simulink model "VTOL_quadplane"  (R2026a)
settings: Solver=ode1  StopTime=120  FixedStep=1/60  MaxStep=0.01
undefined symbols (not defined in the file or in its folder): op_trim, params, Receive, Send
libraries: slpidlib x32, simulink_extras x11, simulink x2, aerolibfltsims x2, aerolibobsolete x1, sim3dlib x1, uavsim3dlib x1
(part 4 of 4)

== system VTOL_quadplane/Autopilot/Height Controller/Subsystem ==
  Constant : Constant  Commented=on  Value=params.trim_Inputs.delta_ele
  Constant1 : Constant  Commented=on  Value=params.trim_Inputs.delta_ail
  From : From  Commented=on  GotoTag=theta_rad  TagVisibility=global
  From1 : From  Commented=on  GotoTag=q_rads  TagVisibility=global
  From2 : From  Commented=on  GotoTag=phi_rad  TagVisibility=global
  From3 : From  Commented=on  GotoTag=p_rads  TagVisibility=global
  PID Controller : slpidlib/PID Controller  Commented=on  Controller=P  Form=Parallel  TimeDomain=Continuous-time  UseExternalTs=off  SampleTime=-1  IntegratorMethod=Forward Euler  FilterMethod=Forward Euler  ControllerParametersSource=internal  P=5.02  I=1  UseKiTs=off  D=0  UseExternalDerivativeSource=off  N=100  UseFilter=on  TunerSelectOption=Transfer Function Based (PID Tuner App)  InitialConditionSource=internal  InitialConditionForIntegrator=0  InitialConditionForFilter=0  DifferentiatorICPrevScaledInput=0  ExternalReset=none  TrackingMode=off  Kt=1  LimitOutput=off  SatLimitsSource=internal  UpperSaturationLimit=inf  LowerSaturationLimit=-inf  LinearizeAsGain=on  AntiWindupMode=none  Kb=1  LimitIntegrator=off  UpperIntegratorSaturationLimit=inf  LowerIntegratorSaturationLimit=-inf  POutMin=[]  POutMax=[]  IOutMin=[]  IOutMax=[]  DOutMin=[]  DOutMax=[]  NOutMin=[]  NOutMax=[]  SumOutMin=[]  SumOutMax=[]  SaturationOutMin=[]  SaturationOutMax=[]  PParamMin=[]  PParamMax=[]  IParamMin=[]  IParamMax=[]  DParamMin=[]  DParamMax=[]  NParamMin=[]  NParamMax=[]  KbParamMin=[]  KbParamMax=[]  KtParamMin=[]  KtParamMax=[]  KbOutMin=[]  KbOutMax=[]  KtOutMin=[]  KtOutMax=[]  IntegratorOutMin=[]  IntegratorOutMax=[]  FilterOutMin=[]  FilterOutMax=[]  SumI1OutMin=[]  SumI1OutMax=[]  SumI2OutMin=[]  SumI2OutMax=[]  SumI3OutMin=[]  SumI3OutMax=[]  SumI4OutMin=[]  SumI4OutMax=[]  SumDOutMin=[]  SumDOutMax=[]  DifferentiatorOutMin=[]  DifferentiatorOutMax=[]  FilterDiffOutCoefMin=[]  FilterDiffOutCoefMax=[]  ReciprocalOutMin=[]  ReciprocalOutMax=[]  SumDenOutMin=[]  SumDenOutMax=[]  SumNumOutMin=[]  SumNumOutMax=[]  DivideOutMin=[]  DivideOutMax=[]  UdiffTsProdOutMin=[]  UdiffTsProdOutMax=[]  NTsProdOutMin=[]  NTsProdOutMax=[]  UintegralTsProdOutMin=[]  UintegralTsProdOutMax=[]  UngainTsProdOutMin=[]  UngainTsProdOutMax=[]  ClampingZeroOutDataTypeStr=Inherit: Inherit via back propagation  ClampingZeroOutMin=[]  ClampingZeroOutMax=[]  FilterDenConstantOutDataTypeStr=Inherit: Inherit via back propagation  FilterDenConstantOutMin=[]  FilterDenConstantOutMax=[]  PCopyOutDataTypeStr=Inherit: Inherit via back propagation  PCopyOutMin=[]  PCopyOutMax=[]  NCopyOutDataTypeStr=Inherit: Inherit via back propagation  NCopyOutMin=[]  NCopyOutMax=[]  IntegratorContinuousStateAttributes=''  IntegratorStateMustResolveToSignalObject=off  IntegratorRTWStateStorageClass=Auto  FilterContinuousStateAttributes=''  FilterStateMustResolveToSignalObject=off  FilterRTWStateStorageClass=Auto  ParallelPVariant=InternalParameters  IdealPVariant=Disabled  IVariant=Disabled  DVariant=Disabled  IntegratorVariant=Disabled  SatVariant=Disabled  AWVariant=Disabled  PCopyVariant=Disabled  TRVariant=Disabled  FdbkBlocksVariant=Forward  IdealPFdbkVariant=Disabled  SatFdbkVariant=Disabled  DerivativeFilterVariant=Disabled  NVariant=Disabled  NCopyVariant=Disabled_SignalSpec  FilterICVariant=Disabled  IntegratorICVariant=Disabled  ExternalResetVariant=Disabled  TRSumVariant=Passthrough  SumFdbkVariant=Disabled  SumVariant=Passthrough_P  TsampFilterVariant=InternalTs  TsampNgainVariant=Passthrough  TsampIntegralVariant=Disabled_SignalSpec  ExternalSaturationOutDataTypeStr=Inherit: Same as second input  DerivativeSourceVariant=Disabled  PreIntVariant=InternalPreInt
  PID Controller1 : slpidlib/PID Controller  Commented=on  Controller=PID  Form=Parallel  TimeDomain=Continuous-time  UseExternalTs=off  SampleTime=-1  IntegratorMethod=Forward Euler  FilterMethod=Forward Euler  ControllerParametersSource=internal  P=-0.189  I=-1.81  UseKiTs=off  D=-0.00495  UseExternalDerivativeSource=off  N=100  UseFilter=on  TunerSelectOption=Transfer Function Based (PID Tuner App)  InitialConditionSource=internal  InitialConditionForIntegrator=0  InitialConditionForFilter=0  DifferentiatorICPrevScaledInput=0  ExternalReset=none  TrackingMode=off  Kt=1  LimitOutput=off  SatLimitsSource=internal  UpperSaturationLimit=inf  LowerSaturationLimit=-inf  LinearizeAsGain=on  AntiWindupMode=none  Kb=1  LimitIntegrator=off  UpperIntegratorSaturationLimit=inf  LowerIntegratorSaturationLimit=-inf  POutMin=[]  POutMax=[]  IOutMin=[]  IOutMax=[]  DOutMin=[]  DOutMax=[]  NOutMin=[]  NOutMax=[]  SumOutMin=[]  SumOutMax=[]  SaturationOutMin=[]  SaturationOutMax=[]  PParamMin=[]  PParamMax=[]  IParamMin=[]  IParamMax=[]  DParamMin=[]  DParamMax=[]  NParamMin=[]  NParamMax=[]  KbParamMin=[]  KbParamMax=[]  KtParamMin=[]  KtParamMax=[]  KbOutMin=[]  KbOutMax=[]  KtOutMin=[]  KtOutMax=[]  IntegratorOutMin=[]  IntegratorOutMax=[]  FilterOutMin=[]  FilterOutMax=[]  SumI1OutMin=[]  SumI1OutMax=[]  SumI2OutMin=[]  SumI2OutMax=[]  SumI3OutMin=[]  SumI3OutMax=[]  SumI4OutMin=[]  SumI4OutMax=[]  SumDOutMin=[]  SumDOutMax=[]  DifferentiatorOutMin=[]  DifferentiatorOutMax=[]  FilterDiffOutCoefMin=[]  FilterDiffOutCoefMax=[]  ReciprocalOutMin=[]  ReciprocalOutMax=[]  SumDenOutMin=[]  SumDenOutMax=[]  SumNumOutMin=[]  SumNumOutMax=[]  DivideOutMin=[]  DivideOutMax=[]  UdiffTsProdOutMin=[]  UdiffTsProdOutMax=[]  NTsProdOutMin=[]  NTsProdOutMax=[]  UintegralTsProdOutMin=[]  UintegralTsProdOutMax=[]  UngainTsProdOutMin=[]  UngainTsProdOutMax=[]  ClampingZeroOutDataTypeStr=Inherit: Inherit via back propagation  ClampingZeroOutMin=[]  ClampingZeroOutMax=[]  FilterDenConstantOutDataTypeStr=Inherit: Inherit via back propagation  FilterDenConstantOutMin=[]  FilterDenConstantOutMax=[]  PCopyOutDataTypeStr=Inherit: Inherit via back propagation  PCopyOutMin=[]  PCopyOutMax=[]  NCopyOutDataTypeStr=Inherit: Inherit via back propagation  NCopyOutMin=[]  NCopyOutMax=[]  IntegratorContinuousStateAttributes=''  IntegratorStateMustResolveToSignalObject=off  IntegratorRTWStateStorageClass=Auto  FilterContinuousStateAttributes=''  FilterStateMustResolveToSignalObject=off  FilterRTWStateStorageClass=Auto  ParallelPVariant=InternalParameters  IdealPVariant=Disabled  IVariant=InternalParameters  DVariant=InternalParameters  IntegratorVariant=Continuous  SatVariant=Disabled  AWVariant=Passthrough  PCopyVariant=Disabled  TRVariant=Disabled  FdbkBlocksVariant=Forward  IdealPFdbkVariant=Disabled  SatFdbkVariant=Disabled  DerivativeFilterVariant=ContFilter  NVariant=InternalParameters  NCopyVariant=Disabled  FilterICVariant=InternalICsFilter  IntegratorICVariant=InternalICs  ExternalResetVariant=Disabled  TRSumVariant=Passthrough  SumFdbkVariant=Disabled  SumVariant=Sum_PID  TsampFilterVariant=InternalTs  TsampNgainVariant=Passthrough  TsampIntegralVariant=Disabled_SignalSpec  ExternalSaturationOutDataTypeStr=Inherit: Same as second input  DerivativeSourceVariant=ErrorSignal  PreIntVariant=InternalPreInt
  PID Controller2 : slpidlib/PID Controller  Commented=on  Controller=P  Form=Parallel  TimeDomain=Continuous-time  UseExternalTs=off  SampleTime=-1  IntegratorMethod=Forward Euler  FilterMethod=Forward Euler  ControllerParametersSource=internal  P=5.02  I=1  UseKiTs=off  D=0  UseExternalDerivativeSource=off  N=100  UseFilter=on  TunerSelectOption=Transfer Function Based (PID Tuner App)  InitialConditionSource=internal  InitialConditionForIntegrator=0  InitialConditionForFilter=0  DifferentiatorICPrevScaledInput=0  ExternalReset=none  TrackingMode=off  Kt=1  LimitOutput=off  SatLimitsSource=internal  UpperSaturationLimit=inf  LowerSaturationLimit=-inf  LinearizeAsGain=on  AntiWindupMode=none  Kb=1  LimitIntegrator=off  UpperIntegratorSaturationLimit=inf  LowerIntegratorSaturationLimit=-inf  POutMin=[]  POutMax=[]  IOutMin=[]  IOutMax=[]  DOutMin=[]  DOutMax=[]  NOutMin=[]  NOutMax=[]  SumOutMin=[]  SumOutMax=[]  SaturationOutMin=[]  SaturationOutMax=[]  PParamMin=[]  PParamMax=[]  IParamMin=[]  IParamMax=[]  DParamMin=[]  DParamMax=[]  NParamMin=[]  NParamMax=[]  KbParamMin=[]  KbParamMax=[]  KtParamMin=[]  KtParamMax=[]  KbOutMin=[]  KbOutMax=[]  KtOutMin=[]  KtOutMax=[]  IntegratorOutMin=[]  IntegratorOutMax=[]  FilterOutMin=[]  FilterOutMax=[]  SumI1OutMin=[]  SumI1OutMax=[]  SumI2OutMin=[]  SumI2OutMax=[]  SumI3OutMin=[]  SumI3OutMax=[]  SumI4OutMin=[]  SumI4OutMax=[]  SumDOutMin=[]  SumDOutMax=[]  DifferentiatorOutMin=[]  DifferentiatorOutMax=[]  FilterDiffOutCoefMin=[]  FilterDiffOutCoefMax=[]  ReciprocalOutMin=[]  ReciprocalOutMax=[]  SumDenOutMin=[]  SumDenOutMax=[]  SumNumOutMin=[]  SumNumOutMax=[]  DivideOutMin=[]  DivideOutMax=[]  UdiffTsProdOutMin=[]  UdiffTsProdOutMax=[]  NTsProdOutMin=[]  NTsProdOutMax=[]  UintegralTsProdOutMin=[]  UintegralTsProdOutMax=[]  UngainTsProdOutMin=[]  UngainTsProdOutMax=[]  ClampingZeroOutDataTypeStr=Inherit: Inherit via back propagation  ClampingZeroOutMin=[]  ClampingZeroOutMax=[]  FilterDenConstantOutDataTypeStr=Inherit: Inherit via back propagation  FilterDenConstantOutMin=[]  FilterDenConstantOutMax=[]  PCopyOutDataTypeStr=Inherit: Inherit via back propagation  PCopyOutMin=[]  PCopyOutMax=[]  NCopyOutDataTypeStr=Inherit: Inherit via back propagation  NCopyOutMin=[]  NCopyOutMax=[]  IntegratorContinuousStateAttributes=''  IntegratorStateMustResolveToSignalObject=off  IntegratorRTWStateStorageClass=Auto  FilterContinuousStateAttributes=''  FilterStateMustResolveToSignalObject=off  FilterRTWStateStorageClass=Auto  ParallelPVariant=InternalParameters  IdealPVariant=Disabled  IVariant=Disabled  DVariant=Disabled  IntegratorVariant=Disabled  SatVariant=Disabled  AWVariant=Disabled  PCopyVariant=Disabled  TRVariant=Disabled  FdbkBlocksVariant=Forward  IdealPFdbkVariant=Disabled  SatFdbkVariant=Disabled  DerivativeFilterVariant=Disabled  NVariant=Disabled  NCopyVariant=Disabled_SignalSpec  FilterICVariant=Disabled  IntegratorICVariant=Disabled  ExternalResetVariant=Disabled  TRSumVariant=Passthrough  SumFdbkVariant=Disabled  SumVariant=Passthrough_P  TsampFilterVariant=InternalTs  TsampNgainVariant=Passthrough  TsampIntegralVariant=Disabled_SignalSpec  ExternalSaturationOutDataTypeStr=Inherit: Same as second input  DerivativeSourceVariant=Disabled  PreIntVariant=InternalPreInt
  PID Controller3 : slpidlib/PID Controller  Commented=on  Controller=PID  Form=Parallel  TimeDomain=Continuous-time  UseExternalTs=off  SampleTime=-1  IntegratorMethod=Forward Euler  FilterMethod=Forward Euler  ControllerParametersSource=internal  P=-0.189  I=-1.81  UseKiTs=off  D=-0.00495  UseExternalDerivativeSource=off  N=100  UseFilter=on  TunerSelectOption=Transfer Function Based (PID Tuner App)  InitialConditionSource=internal  InitialConditionForIntegrator=0  InitialConditionForFilter=0  DifferentiatorICPrevScaledInput=0  ExternalReset=none  TrackingMode=off  Kt=1  LimitOutput=off  SatLimitsSource=internal  UpperSaturationLimit=inf  LowerSaturationLimit=-inf  LinearizeAsGain=on  AntiWindupMode=none  Kb=1  LimitIntegrator=off  UpperIntegratorSaturationLimit=inf  LowerIntegratorSaturationLimit=-inf  POutMin=[]  POutMax=[]  IOutMin=[]  IOutMax=[]  DOutMin=[]  DOutMax=[]  NOutMin=[]  NOutMax=[]  SumOutMin=[]  SumOutMax=[]  SaturationOutMin=[]  SaturationOutMax=[]  PParamMin=[]  PParamMax=[]  IParamMin=[]  IParamMax=[]  DParamMin=[]  DParamMax=[]  NParamMin=[]  NParamMax=[]  KbParamMin=[]  KbParamMax=[]  KtParamMin=[]  KtParamMax=[]  KbOutMin=[]  KbOutMax=[]  KtOutMin=[]  KtOutMax=[]  IntegratorOutMin=[]  IntegratorOutMax=[]  FilterOutMin=[]  FilterOutMax=[]  SumI1OutMin=[]  SumI1OutMax=[]  SumI2OutMin=[]  SumI2OutMax=[]  SumI3OutMin=[]  SumI3OutMax=[]  SumI4OutMin=[]  SumI4OutMax=[]  SumDOutMin=[]  SumDOutMax=[]  DifferentiatorOutMin=[]  DifferentiatorOutMax=[]  FilterDiffOutCoefMin=[]  FilterDiffOutCoefMax=[]  ReciprocalOutMin=[]  ReciprocalOutMax=[]  SumDenOutMin=[]  SumDenOutMax=[]  SumNumOutMin=[]  SumNumOutMax=[]  DivideOutMin=[]  DivideOutMax=[]  UdiffTsProdOutMin=[]  UdiffTsProdOutMax=[]  NTsProdOutMin=[]  NTsProdOutMax=[]  UintegralTsProdOutMin=[]  UintegralTsProdOutMax=[]  UngainTsProdOutMin=[]  UngainTsProdOutMax=[]  ClampingZeroOutDataTypeStr=Inherit: Inherit via back propagation  ClampingZeroOutMin=[]  ClampingZeroOutMax=[]  FilterDenConstantOutDataTypeStr=Inherit: Inherit via back propagation  FilterDenConstantOutMin=[]  FilterDenConstantOutMax=[]  PCopyOutDataTypeStr=Inherit: Inherit via back propagation  PCopyOutMin=[]  PCopyOutMax=[]  NCopyOutDataTypeStr=Inherit: Inherit via back propagation  NCopyOutMin=[]  NCopyOutMax=[]  IntegratorContinuousStateAttributes=''  IntegratorStateMustResolveToSignalObject=off  IntegratorRTWStateStorageClass=Auto  FilterContinuousStateAttributes=''  FilterStateMustResolveToSignalObject=off  FilterRTWStateStorageClass=Auto  ParallelPVariant=InternalParameters  IdealPVariant=Disabled  IVariant=InternalParameters  DVariant=InternalParameters  IntegratorVariant=Continuous  SatVariant=Disabled  AWVariant=Passthrough  PCopyVariant=Disabled  TRVariant=Disabled  FdbkBlocksVariant=Forward  IdealPFdbkVariant=Disabled  SatFdbkVariant=Disabled  DerivativeFilterVariant=ContFilter  NVariant=InternalParameters  NCopyVariant=Disabled  FilterICVariant=InternalICsFilter  IntegratorICVariant=InternalICs  ExternalResetVariant=Disabled  TRSumVariant=Passthrough  SumFdbkVariant=Disabled  SumVariant=Sum_PID  TsampFilterVariant=InternalTs  TsampNgainVariant=Passthrough  TsampIntegralVariant=Disabled_SignalSpec  ExternalSaturationOutDataTypeStr=Inherit: Same as second input  DerivativeSourceVariant=ErrorSignal  PreIntVariant=InternalPreInt
  Saturation1 : Saturate  Commented=on  UpperLimit=deg2rad(25)  LowerLimit=-deg2rad(25)
  Saturation3 : Saturate  Commented=on  UpperLimit=deg2rad(25)  LowerLimit=-deg2rad(25)
  Sum{,1,4..5} (4 alike) : Sum  Commented=on  Inputs=|+-
  Sum3 : Sum  Commented=on  Inputs=++|
  Sum6 : Sum  Commented=on  Inputs=++|
  Transfer Fcn : TransferFcn  Commented=on  Denominator=[0.02 1]
  Transfer Fcn1 : TransferFcn  Commented=on  Denominator=[0.02 1]
  wires:
  Sum/1 -> PID Controller/1
  Saturation3/1 -> Sum4/1
  Saturation1/1 -> Sum/1
  Sum6/1 -> Transfer Fcn1/1
  PID Controller1/1 -> Sum3/2
  PID Controller2/1 -> Sum5/1
  Transfer Fcn1/1 -> ?
  From/1 -> Sum/2
  Constant/1 -> Sum3/1
  Transfer Fcn/1 -> ?
  From2/1 -> Sum4/2
  From3/1 -> Sum5/2
  Sum4/1 -> PID Controller2/1
  From1/1 -> Sum1/2
  Sum3/1 -> Transfer Fcn/1
  PID Controller3/1 -> Sum6/2
  Sum5/1 -> PID Controller3/1
  ? -> Saturation1/1
  PID Controller/1 -> Sum1/1
  ? -> Saturation3/1
  Constant1/1 -> Sum6/1
  Sum1/1 -> PID Controller1/1

== matlab function VTOL_quadplane/MATLAB Function1 ==
  settings: updateMethod=DISCRETE
  data: cruise_speed input; lambda output; mc_forward_speed output; cruise_altitude input; mc_speed input; speed input; height input; transition_speed input; mc_height output; fw_speed output; fw_height output; mode output; transition_height input
function [lambda, mc_forward_speed, mc_height, fw_speed, fw_height, mode] = mode_manager( ...
    cruise_speed, cruise_altitude, mc_speed, speed, height, transition_speed, transition_height)
%MODE_MANAGER  VTOL quadplane mission state machine.
%
%   0 = climb straight to transition_height
%   1 = hover at transition_height for HOVER_TIME before transitioning
%   2 = TRANSITION: lambda ramps 0->1, forward-speed target ramps 0->
%       transition_speed, AND altitude ramps transition_height->
%       cruise_altitude - ALL CONTINUOUSLY, no step inputs to any
%       controller, so nothing gets a derivative kick.
%   3 = COMPLETE FW: only entered once lambda has reached 1, the aircraft
%       has reached cruise_altitude, AND transition_speed has been
%       reached. MC path is given no active target here.

    persistent state timer lambda_state climb_timer speed_timer
    if isempty(state)
        state       = 0;
        timer       = 0;
        lambda_state = 0;
        climb_timer  = 0;
        speed_timer  = 0;
    end

    DT              = 1/100;  % [s] model's fixed step = 1/simulation time
    HOVER_TIME      = 0.5;    % [s] wait at transition altitude before ramping
    T_LAMBDA_RAMP   = 20.0;   % [s] total time for lambda to go 0->1, smoothly
    ALT_CLIMB_TIME  = 10.0;   % [s] time to climb from transition_height to cruise_altitude
    SPEED_RAMP_TIME = 5.0;   % [s] time to ramp forward-speed target to transition_speed
                              % (feeds the pitch PID - must NOT be a step)

    alt_target   = transition_height;  % defaults so they're defined on every path
    speed_target = 0;

    % ---- state transitions ----
    if state == 0 && height <= transition_height + 0.5
        state = 1;
        timer = 0;
    end

    if state == 1
        timer = timer + DT;
        if timer >= HOVER_TIME
            state       = 2;
            timer       = 0;
            climb_timer = 0;   % start all ramps together
            speed_timer = 0;
        end
    end

    if state == 2
        % ---- lambda ramp: smooth, continuous, no steps ----
        lambda_state = min(lambda_state + DT / T_LAMBDA_RAMP, 1);

        % ---- altitude ramp (smoothstep - no rate discontinuity) ----
        climb_timer = climb_timer + DT;
        fa = min(climb_timer / ALT_CLIMB_TIME, 1);
        sa = 3*fa^2 - 2*fa^3;
        alt_target = transition_height + sa * (cruise_altitude - transition_height);

        % ---- forward-speed ramp (smoothstep - no step into the PID) ----
        speed_timer = speed_timer + DT;
        fs = min(speed_timer / SPEED_RAMP_TIME, 1);
        ss = 3*fs^2 - 2*fs^3;
        speed_target = ss * transition_speed;

        % only lock into complete FW once ALL three are true
        if lambda_state >= 1 && height <= cruise_altitude + 0.5 && speed >= transition_speed
            state = 3;
        end
    end

    % ---- outputs ----
    if state == 0 || state == 1
        mc_forward_speed = 0;
        fw_speed         = 0;
        mc_height        = transition_height;
        fw_height        = transition_height;

    elseif state == 2
        mc_forward_speed = speed_target;   % ramped, not stepped
        fw_speed         = speed_target;
        mc_height        = alt_target;
        fw_height        = alt_target;

    else % state == 3 - complete FW, MC path given nothing to chase
        mc_forward_speed = 0;
        mc_height        = height;        % freeze - zero error, no MC climb command
        fw_speed         = cruise_speed;
        fw_height        = cruise_altitude;
    end

    lambda = lambda_state;
    mode   = state;
end

== matlab function VTOL_quadplane/MATLAB Function3 ==
  settings: updateMethod=DISCRETE
  data: cruise_speed input; lambda output; mc_forward_speed output; cruise_altitude input; mc_speed input; speed input; height input; transition_speed input; mc_height output; fw_speed output; fw_height output; mode output; transition_height input
function [lambda, mc_forward_speed, mc_height, fw_speed, fw_height, mode] = mode_manager( ...
    cruise_speed, cruise_altitude, mc_speed, speed, height, transition_speed, transition_height)

    persistent state hover_timer
    if isempty(state)
        state       = 0;   % 0 = climb, 1 = hover, 2 = transition/cruise
        hover_timer = 0;
    end

    DT         = 1/60;  % [s] model's fixed step
    HOVER_TIME = 5.0;   % [s]

    if state == 0 && height <= transition_height + 2
        state       = 1;
        hover_timer = 0;
    end

    if state == 1
        hover_timer = hover_timer + DT;
        if hover_timer >= HOVER_TIME
            state = 2;
        end
    end

    if state == 0 || state == 1
        mc_forward_speed = 0;
        mc_height        = transition_height;
        fw_speed         = 0;
        fw_height        = transition_height;
        lambda           = 0;
    else
        mc_forward_speed = cruise_speed;
        mc_height        = transition_height;
        fw_speed         = cruise_speed;
        fw_height        = transition_height;
        lambda           = 1;
    end

    mode = state;
end

== matlab function VTOL_quadplane/MATLAB Function4 ==
  settings: updateMethod=DISCRETE
  data: cruise_speed input; lambda output; mc_forward_speed output; cruise_altitude input; mc_speed input; speed input; height input; transition_speed input; mc_height output; fw_speed output; fw_height output; mode output; transition_height input
function [lambda, mc_forward_speed, mc_height, fw_speed, fw_height, mode] = mode_manager( ...
    cruise_speed, cruise_altitude, mc_speed, speed, height, transition_speed, transition_height)

    persistent state hover_timer lambda_state
    if isempty(state)
        state        = 0;   % 0 = climb, 1 = hover, 2 = transition/cruise
        hover_timer  = 0;
        lambda_state = 0;
    end

    DT         = 1/60;  % [s] model's fixed step
    HOVER_TIME = 5.0;   % [s]
    T_BLEND    = 6.0;   % [s] time for lambda to ramp 0 -> 1 - raise this
                        % to make the transition even gentler

    if state == 0 && height <= transition_height + 2
        state       = 1;
        hover_timer = 0;
    end

    if state == 1
        hover_timer = hover_timer + DT;
        if hover_timer >= HOVER_TIME
            state = 2;
        end
    end

    if state == 0 || state == 1
        mc_forward_speed = 0;
        mc_height        = transition_height;
        fw_speed         = 0;
        fw_height        = transition_height;
        lambda_state     = 0;
    else
        mc_forward_speed = cruise_speed;
        mc_height        = transition_height;
        fw_speed         = cruise_speed;
        fw_height        = transition_height;
        lambda_state     = min(lambda_state + DT / T_BLEND, 1);
    end

    lambda = lambda_state;
    mode   = state;
end

== matlab function VTOL_quadplane/MATLAB Function5 ==
  settings: updateMethod=DISCRETE
  data: cruise_speed input; lambda output; mc_forward_speed output; cruise_altitude input; mc_speed input; speed input; height input; transition_speed input; mc_height output; fw_speed output; fw_height output; mode output; transition_height input
function [lambda, mc_forward_speed, mc_height, fw_speed, fw_height, mode] = mode_manager( ...
    cruise_speed, cruise_altitude, mc_speed, speed, height, transition_speed, transition_height)

    persistent state timer lambda_state
    if isempty(state)
        state        = 0;   % 0 = climb, 1 = hover, 2 = ramp, 3 = cruise
        timer        = 0;
        lambda_state = 0;
    end

    DT         = 1/60;  % [s] model's fixed step
    HOVER_TIME = 5.0;   % [s] wait at transition altitude before ramping
    STEP_TIME  = 2.0;   % [s] between each 0.1 increment (10 steps x 1s = 10s)

    % ---- state transitions ----
    if state == 0 && height <= transition_height + 0.5
        state = 1;
        timer = 0;
    end

    if state == 1
        timer = timer + DT;
        if timer >= HOVER_TIME
            state = 2;
            timer = 0;
        end
    end

    if state == 2
        timer = timer + DT;
        if timer >= STEP_TIME
            timer        = 0;
            lambda_state = lambda_state + 0.1;
        end
        if lambda_state >= 1
            lambda_state = 1;
            state        = 3;
        end
    end

    if speed >= transition_speed
        lambda_state = 1;
        state        = 3;
    end

    % ---- outputs ----
    if state == 0 || state == 1
        mc_forward_speed = 0;
        fw_speed         = 0;
    else
        mc_forward_speed = cruise_speed;
        fw_speed         = cruise_speed;
    end

    mc_height = transition_height;
    fw_height = transition_height;
    lambda    = lambda_state;
    mode      = state;
end

== matlab function VTOL_quadplane/MATLAB Function6 ==
  settings: updateMethod=DISCRETE
  data: cruise_speed input; lambda output; mc_forward_speed output; cruise_altitude input; mc_speed input; speed input; height input; transition_speed input; mc_height output; fw_speed output; fw_height output; mode output; transition_height input
function [lambda, mc_forward_speed, mc_height, fw_speed, fw_height, mode] = mode_manager( ...
    cruise_speed, cruise_altitude, mc_speed, speed, height, transition_speed, transition_height)

    persistent state timer lambda_state
    if isempty(state)
        state        = 0;   % 0 = climb, 1 = hover, 2 = ramp, 3 = cruise
        timer        = 0;
        lambda_state = 0;
    end

    DT         = 1/600;  % [s] model's fixed step
    HOVER_TIME = 2.0;   % [s] wait at transition altitude before ramping
    STEP_TIME  = 1.0;   % [s] between each 0.1 increment (10 steps x 1s = 10s)

    % ---- state transitions ----
    if state == 0 && height <= transition_height + 0.5
        state = 1;
        timer = 0;
    end

    if state == 1
        timer = timer + DT;
        if timer >= HOVER_TIME
            state = 2;
            timer = 0;
        end
    end

    if state == 2
        timer = timer + DT;
        if timer >= STEP_TIME
            timer        = 0;
            lambda_state = lambda_state + 0.1;
        end
        if lambda_state >= 1
            lambda_state = 1;
            state        = 3;
        end
    end

    if speed >= transition_speed
        lambda_state = 1;
        state        = 3;
    end

    % ---- outputs ----
    if state == 0 || state == 1
        mc_forward_speed = 0;
        fw_speed         = 0;
    else
        mc_forward_speed = cruise_speed;
        fw_speed         = cruise_speed;
    end

    mc_height = transition_height;
    fw_height = transition_height;
    lambda    = lambda_state;
    mode      = state;
end

== matlab function VTOL_quadplane/MATLAB Function7 ==
  settings: updateMethod=DISCRETE
  data: cruise_speed input; lambda output; mc_forward_speed output; cruise_altitude input; mc_speed input; speed input; height input; transition_speed input; mc_height output; fw_speed output; fw_height output; mode output; transition_height input
function [lambda, mc_forward_speed, mc_height, fw_speed, fw_height, mode] = mode_manager( ...
    cruise_speed, cruise_altitude, mc_speed, speed, height, transition_speed, transition_height)

    persistent state timer lambda_state
    if isempty(state)
        state        = 0;   % 0 = climb, 1 = hover, 2 = ramp, 3 = cruise
        timer        = 0;
        lambda_state = 0;
    end

    DT         = 1/600;  % [s] model's fixed step
    HOVER_TIME = 0.5;   % [s] wait at transition altitude before ramping
    STEP_TIME  = 3.0;   % [s] between each 0.1 increment (10 steps x 1s = 10s)

    % ---- state transitions ----
    if state == 0 && height <= transition_height + 0.5
        state = 1;
        timer = 0;
    end

    if state == 1
        timer = timer + DT;
        if timer >= HOVER_TIME
            state = 2;
            timer = 0;
        end
    end

    if state == 2
        timer = timer + DT;
        if timer >= STEP_TIME
            timer        = 0;
            lambda_state = lambda_state + 0;
        end
        if lambda_state >= 1
            lambda_state = 1;
            state        = 3;
        end
    end

    if speed >= transition_speed
        lambda_state = 1+0;
        state        = 3;
    end

    % ---- outputs ----
    if state == 0 || state == 1
        mc_forward_speed = 0;
        fw_speed         = 0;
    else
        mc_forward_speed = cruise_speed;
        fw_speed         = cruise_speed;
        fw_height        = cruise_altitude;
    end

    mc_height = transition_height;
    fw_height = cruise_altitude;
    lambda    = lambda_state;
    mode      = state;
end

== matlab function VTOL_quadplane/Pusher Forces and Moments ==
  data: u input; F_fw output; M_fw output; params input
function [F_fw, M_fw] = pusher_forces_and_moments(u, params)


% Function to commute forces and moments contributed by the pusher motor
% FW_propulsion_data;
% Extracting appriopriate input
delta_T = u(1); % Throttle Input

% Thrust generated by pusher motor
T_pusher = interp1(params.fw.Throttle, params.fw.Thrust, delta_T, 'linear', 'extrap');
Q_pusher = interp1(params.fw.Throttle, params.fw.Torque, delta_T, 'linear', 'extrap');

% Clamp to zero to avoid negative thrust
T_pusher = max(T_pusher, 0);
Q_pusher = max(Q_pusher, 0);

F_fw = [T_pusher; 0 ; 0];    
% F_fw = F_fw';

% Moments generated by pusher motor
r_pusher = [0;0;0]; % pusher position


% Moment computation
% M_fw = cross(F_fw, r_pusher);
M_fw = cross(r_pusher, F_fw) + [Q_pusher; 0; 0];

% % M_fw = M';% + [Q_pusher, 0, 0];

end

== matlab function VTOL_quadplane/Motor Mixing/MATLAB Function ==
  data: Throttle input; sigma_1 output; roll input; pitch input; yaw input; sigma_2 output; sigma_3 output; sigma_4 output
function [sigma_1, sigma_2, sigma_3, sigma_4] = Motor_mapping(Throttle, roll, pitch, yaw)

Mix_mat = [1 , -1,  1,  1;
           1,   1, -1,  1;
           1,   1,  1, -1;
           1,  -1, -1, -1]; 

Inputs = [Throttle; roll; pitch; yaw]; %User inputs

sigma = Mix_mat*Inputs;

sigma_1 = sigma(1,:);
sigma_2 = sigma(2,:);
sigma_3 = sigma(3,:);
sigma_4 = sigma(4,:);

end

== matlab function VTOL_quadplane/Autopilot/MATLAB Function ==
  data: theta_c input; del_e output; theta input; q input; Va input; params input; zeta_theta input; theta_e_max input; delta_e_max input; kp_theta output; kd_theta output; omega_n_theta output; K_theta_DC output
function [del_e, kp_theta, kd_theta, omega_n_theta, K_theta_DC] = ...
    pitch_attitude_controller(theta_c, theta, q, Va, params, zeta_theta, theta_e_max, delta_e_max)
%PITCH_ATTITUDE_CONTROLLER  Pitch-attitude-hold autopilot (elevator channel).
%
%   Implements the successive-loop-closure pitch attitude hold loop from
%   Beard & McLain, "Small Unmanned Aircraft," Ch. 6, Sec. 6.4.1
%   (Fig. 6.15, Eqs. 6.18-6.23), using the a_theta1..a_theta3 coefficients
%   from Ch. 5 (Sec. 5.5) and the airframe parameters produced by Params1.m.
%
%   [del_e, kp_theta, kd_theta, omega_n_theta, K_theta_DC] = ...
%       pitch_attitude_controller(theta_c, theta, q, Va, params, ...
%                                  zeta_theta, theta_e_max, delta_e_max)
%
% INPUTS
%   theta_c      - commanded pitch angle                        [rad]
%   theta        - current pitch angle                          [rad]
%   q            - body-axis pitch rate                         [rad/s]
%   Va           - airspeed at which a_theta1..3 are evaluated  [m/s]
%                  (use the trim/nominal airspeed for a fixed-gain
%                  design, per the book; pass the instantaneous
%                  airspeed instead if you want simple gain scheduling)
%   params       - aircraft parameter struct from Params1.m
%   zeta_theta   - desired pitch-loop damping ratio (design choice, e.g. 0.707)
%   theta_e_max  - maximum expected pitch error, used to size kp_theta [rad]
%   delta_e_max  - elevator actuator saturation limit                 [rad]
%
% OUTPUTS
%   del_e          - commanded elevator deflection [rad], saturated to
%                    +/- delta_e_max
%   kp_theta       - proportional gain                 (Eq. 6.?, ahead of 6.19)
%   kd_theta       - derivative (rate) gain             (Eq. 6.22)
%   omega_n_theta  - resulting pitch-loop natural frequency (Eq. 6.21)
%   K_theta_DC     - inner-loop DC gain, theta -> theta_c (Eq. 6.23),
%                    needed by the outer altitude/airspeed-from-pitch loops
%
%   Note: kp_theta, kd_theta, omega_n_theta and K_theta_DC only depend on
%   Va and params/tuning choices, not on theta_c/theta/q. If you are
%   calling this every simulation step with a fixed Va, you are free to
%   compute the gains once offline and hard-code them instead.

% ---- unpack the physical parameters needed for a_theta1..3 ----
rho = params.constants.rho;      % air density                [kg/m^3]
c   = params.geometric.c;        % mean aerodynamic chord     [m]
S   = params.geometric.S;        % wing area                  [m^2]
Jy  = params.geometric.I_y;      % pitch moment of inertia    [kg.m^2]

Cm_alpha = params.aero.Cm_alpha; % pitching-moment slope wrt alpha
Cm_q     = params.aero.Cm_q;     % pitching-moment slope wrt pitch rate
Cm_de    = params.aero.Cm_de;    % pitching-moment slope wrt elevator

% ---- longitudinal short-period coefficients (Ch.5, Sec 5.5) ----
a_theta1 = -(rho*Va^2*c*S)/(2*Jy) * Cm_q * (c/(2*Va));
a_theta2 = -(rho*Va^2*c*S)/(2*Jy) * Cm_alpha;
a_theta3 =  (rho*Va^2*c*S)/(2*Jy) * Cm_de;

% ---- pitch-loop gain design (Eqs. 6.19-6.23) ----
kp_theta      = (delta_e_max/theta_e_max) * sign(a_theta3);
omega_n_theta = sqrt(a_theta2 + (delta_e_max/theta_e_max)*abs(a_theta3));
kd_theta      = (2*zeta_theta*omega_n_theta - a_theta1) / a_theta3;
K_theta_DC    = (kp_theta*a_theta3) / (a_theta2 + kp_theta*a_theta3);

% ---- pitch attitude-hold control law (output of the pitch loop) ----
del_e_unsat = kp_theta*(theta_c - theta) - kd_theta*q;

% ---- elevator actuator saturation ----
del_e = max(min(del_e_unsat, delta_e_max), -delta_e_max);

end

== matlab function VTOL_quadplane/Motor Mixing/MATLAB Function1 ==
  data: u input; Omega_1 output; Throttle input; Omega_2 output; RPM input; Omega_3 output; Omega_4 output
function [Omega_1, Omega_2, Omega_3, Omega_4] = RPM_from_throttle_percentage(u,Throttle, RPM)


% NED frame
% Extracting control inputs
sigma1       = u(1); % Rotor 1 Throttle %
sigma2       = u(2); % Rotor 2 Throttle %
sigma3       = u(3); % Rotor 3 Throttle %
sigma4       = u(4); % Rotor 4 Throttle %

% % Motor Positioning
% % [M1:FR, M2:FL, M3:RL, M4:RR]
% % spin direction = [CW:+1, CCW:-1]
% % Extracting motor positions
% r1 = params.prop.r1(:); %FR-CCW
% r2 = params.prop.r2(:); %RL-CCW
% r3 = params.prop.r3(:); %FL-CW
% r4 = params.prop.r4(:); %RR-CW

% throttle to RPM mapping
W1       = interp1(Throttle, RPM, sigma1, 'linear','extrap');
Omega_1  = (W1*2*pi/60)^2;

W2       = interp1(Throttle, RPM, sigma2, 'linear','extrap');
Omega_2  = (W2*2*pi/60)^2;

W3       = interp1(Throttle, RPM, sigma3, 'linear','extrap');
Omega_3  = (W3*2*pi/60)^2;

W4       = interp1(Throttle, RPM, sigma4, 'linear','extrap');
Omega_4  = (W4*2*pi/60)^2;

end

== matlab function VTOL_quadplane/Motor Mixing/MATLAB Function2 ==
  data: omega input; F_vtol output; c_T input; M_vtol output; c_M input
function [F_vtol, M_vtol] = vertical_forces_and_moments(omega, c_T, c_M)


% NED frame
% Extracting control inputs
omega1       = omega(1); % Rotor 1 Throttle %
omega2       = omega(2); % Rotor 2 Throttle %
omega3       = omega(3); % Rotor 3 Throttle %
omega4       = omega(4); % Rotor 4 Throttle %

% Constants
theta = 49.76; % angle between motor arm and x-y plane
d = 0.815; % arm length

% angles from +X axis to arm lengths
a_1 = 90 - theta;
a_4 = 90 + theta;
a_2 = 180 + (90 - theta);
a_3 = 270 + theta;

% M1 = [c_T; d*c_T*cosd(theta); d*c_T*sind(theta); c_M];

M1 = [c_T; -d*c_T; d*c_T; c_M];


 % M2 = [ omega1, omega2,   omega3,   omega4;
 %        -omega1, omega2,  omega3,  -omega4;
 %        omega1, -omega2,  omega3,   -omega4;
 %        omega1, omega2,  -omega3,  -omega4 ]; 

M2 = [ omega1,                     omega2,            omega3,            omega4;
       sind(a_1)*omega1, sind(a_2)*omega2,  sind(a_3)*omega3,  sind(a_4)*omega4;
       cosd(a_1)*omega1, cosd(a_2)*omega2,  cosd(a_3)*omega3,  cosd(a_4)*omega4;
       omega1,                     omega2,           -omega3,           -omega4]; 


F_M = M1.*M2;

F_vtol = [0; 0; -sum(F_M(1,:))];

M_vtol = [sum(F_M(2,:));
          sum(F_M(3,:));
          sum(F_M(4,:))];

end

== matlab function VTOL_quadplane/MATLAB Function2 ==
  settings: updateMethod=DISCRETE
  data: cruise_speed input; lambda output; mc_forward_speed output; cruise_altitude input; mc_speed input; speed input; height input; transition_speed input; mc_height output; fw_speed output; fw_height output; mode output; transition_height input
function [lambda, mc_forward_speed, mc_height, fw_speed, fw_height, mode] = mode_manager( ...
    cruise_speed, cruise_altitude, mc_speed, speed, height, transition_speed, transition_height)

    persistent state
    if isempty(state)
        state = 0;   % 0 = climb, 1 = transition/cruise
    end

    if state == 0 && height <= transition_height + 2
        state = 1;
    end

    if state == 0
        mc_forward_speed = 0;
        mc_height        = transition_height;
        fw_speed         = 0;
        fw_height        = transition_height;
        lambda           = 0;
    else
        mc_forward_speed = cruise_speed;
        mc_height        = transition_height;
        fw_speed         = cruise_speed;
        fw_height        = transition_height;
        lambda           = 1;
    end

    mode = state;
end
